simulink model "ACC_linear"  (Simulink 9.2)
settings: Solver=ode45  StartTime=0.0  StopTime=15  RelTol=1e-6
settings Model: Creator=jinwooro  LastModifiedBy=jinwooro
settings DataIOCC: LimitDataPoints=off  SaveFormat=Dataset  SignalLoggingSaveFormat=Dataset
settings OptimizationCC: LifeSpan=auto
settings DebuggingCC: UnderspecifiedInitializationDetection=Simplified  MergeDetectMultiDrivingBlocksExec=error  FcnCallInpInsideContextMsg=error  StateNameClashWarn=none  SFUnexpectedBacktrackingDiag=error  SFNoUnconditionalDefaultTransitionDiag=error  SFExecutionAtInitializationDiag=warning
settings HardwareCC: ProdBitPerPointer=64  ProdBitPerSizeT=64  ProdBitPerPtrDiffT=64  ProdLargestAtomicFloat=Float  ProdIntDivRoundTo=Zero  ProdEndianess=LittleEndian  ProdWordSize=64  ProdHWDeviceType=Intel->x86-64 (Windows64)
settings ModelReferenceCC: PropagateSignalLabelsOutOfModel=on
settings SFSimCC: SimUseLocalCustomCode=on
settings RTWCC: RTWUseLocalCustomCode=on
settings CodeAppCC: StateflowObjectComments=off
settings GRTTargetCC: TargetLangStandard=C99 (ISO)  GeneratePreprocessorConditionals=Use local settings  CombineOutputUpdateFcns=on  GRTInterface=off
settings ConfigComp: CovMetricSettings=dwe  CovHtmlReporting=off  CovSaveCumulativeToWorkspaceVar=off  CovSaveSingleToWorkspaceVar=off  CovExternalEMLEnable=on

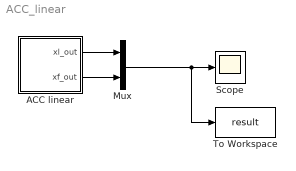
== system ACC_linear ==
  ACC linear : Stateflow chart  TreatAsAtomicUnit=on
  Mux : Mux  Inputs=2
  Scope : Scope
  To Workspace : ToWorkspace  VariableName=result  SaveFormat=Timeseries  SampleTime=-1
  wires:
  ACC linear/1(xl_out) -> Mux/1
  ACC linear/2(xf_out) -> Mux/2
  Mux/1 -> To Workspace/1, Scope/1

== stateflow chart ACC linear ==
  settings: updateMethod=CONTINUOUS
  state Driving
    du:
    tau_dot = 1;
    xl_dot = 7 * sin(0.5 * tau) + 7;
    xf_dot = (xl - xf);
    xl_out = xl;
    xf_out = xf;
  state Collision
    du:
    tau_dot = 1;
    xl_dot = 0;
    xf_dot = 0;
    xf_out = xf;
    xl_out = xl;
  (default) -> Driving : {
      | xl = 15;
      | xf = 0;
      | tau = 0;
      | }
  Driving -> Collision : [power(xl - xf - 5, 0.5) <= 0]
  data: xf local double; xl_out output double; tau local double; xl local double; xf_out output double
  data xf settings: updateMethod=SF_CONTINUOUS_TIME_DATA
  data tau settings: updateMethod=SF_CONTINUOUS_TIME_DATA
  data xl settings: updateMethod=SF_CONTINUOUS_TIME_DATA
